simulink model "微分2"  (R2018b)
settings: Solver=VariableStepAuto  StartTime=0.0  StopTime=10.0  RelTol=1e-3
settings Model: Creator=Jason  LastModifiedBy=Jason

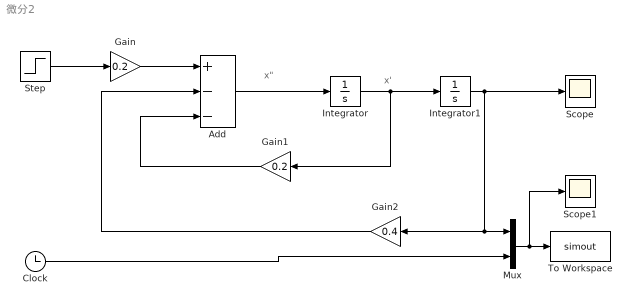
== system 微分2 ==
  note: x'
  note: x"
  Add : Sum  Inputs=+--
  Clock : Clock
  Gain : Gain  Gain=0.2
  Gain1 : Gain  Gain=0.2
  Gain2 : Gain  Gain=0.4
  Integrator : Integrator
  Integrator1 : Integrator
  Mux : Mux  Inputs=2
  Scope : Scope
  Scope1 : Scope
  Step : Step  SampleTime=0
  To Workspace : ToWorkspace  VariableName=simout  SaveFormat=Timeseries  SampleTime=-1
  wires:
  Step/1 -> Gain/1
  Gain/1 -> Add/1
  Add/1 -> Integrator/1
  Integrator/1 -> Gain1/1, Integrator1/1
  Integrator1/1 -> Mux/1, Gain2/1, Scope/1
  Gain1/1 -> Add/3
  Gain2/1 -> Add/2
  Clock/1 -> Mux/2
  Mux/1 -> Scope1/1, To Workspace/1
